simulink model "FIR_Filter"  (R2020a)
settings: Solver=FixedStepAuto  StartTime=0.0  StopTime=10.0  FixedStep=0.2  RelTol=1e-3
settings Model: Creator=user  LastModifiedBy=user
settings DataIOCC: SaveOutput=off  SaveTime=off

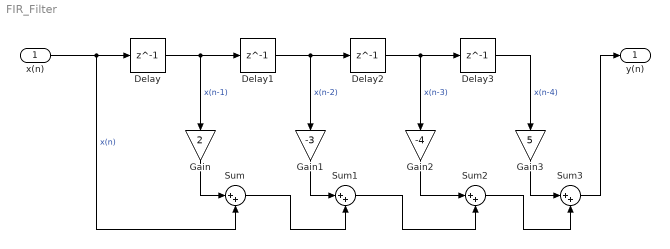
== system FIR_Filter ==
  x(n) : Inport  OutDataTypeStr=double  PortDimensions=1  SampleTime=[0.20000000000000001,0]
  Delay{,1..3} (4 alike) : Delay  DelayLength=1
  Gain : Gain  Gain=2
  Gain1 : Gain  Gain=-3
  Gain2 : Gain  Gain=-4
  Gain3 : Gain  Gain=5
  Sum{,1..3} (4 alike) : Sum  Inputs=|++
  y(n) : Outport  OutDataTypeStr=double  PortDimensions=1  SampleTime=[0.20000000000000001,0]
  wires:
  Delay1/1 -> Delay2/1, Gain1/1  "x(n-2)"
  Gain3/1 -> Sum3/1
  Delay/1 -> Delay1/1, Gain/1  "x(n-1)"
  Delay3/1 -> Gain3/1  "x(n-4)"
  x(n)/1 -> Delay/1, Sum/2  "x(n)"
  Sum2/1 -> Sum3/2
  Gain1/1 -> Sum1/1
  Sum1/1 -> Sum2/2
  Gain2/1 -> Sum2/1
  Delay2/1 -> Delay3/1, Gain2/1  "x(n-3)"
  Gain/1 -> Sum/1
  Sum/1 -> Sum1/2
  Sum3/1 -> y(n)/1
